simulink model "Fig134"  (R2014a)
settings: Solver=FixedStepDiscrete  StartTime=0.0  StopTime=.05  FixedStep=1.25e-6  RelTol=1e-3
undefined symbols (not defined in the file): fdesignblkfcn, gcbh
libraries: commchan3 x1, commanapbnd3 x1
(part 1 of 2)
settings Model: Creator=Dennis Silage  LastModifiedBy=Silage
settings SolverCC: AutoInsertRateTranBlk=on
settings DataIOCC: SignalLoggingSaveFormat=ModelDataLogs
settings OptimizationCC: ExpressionDepthLimit=2147483647  InitFltsAndDblsToZero=on
settings DebuggingCC: UnderspecifiedInitializationDetection=Classic  FcnCallInpInsideContextMsg=UseLocalSettings  StateNameClashWarn=warning
settings GRTTargetCC: CombineOutputUpdateFcns=off  GRTInterface=on

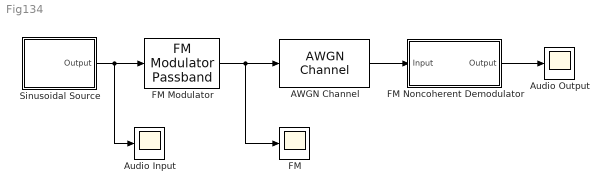
== system Fig134 ==
  AWGN Channel : commchan3/AWGN Channel  InputProcessing=Inherited (this choice will be removed - see release notes)  seed=randseed  noiseMode=Variance from mask  EbNodB=10  EsNodB=10  SNRdB=10  bitsPerSym=1  Ps=1  Tsym=1  variance=0
  Audio Output : Scope
      settings: TimeRange=0.01  MaxDataPoints=8000
  Audio Input : Scope
      settings: TimeRange=0.01  YMin=-2  YMax=2  SaveName=ScopeData2  MaxDataPoints=8000
  FM : Scope
      settings: TimeRange=0.01  MaxDataPoints=8000
  FM Modulator : commanapbnd3/FM Modulator Passband  Fc=20000  Ph=0  Kc=500
  FM Noncoherent Demodulator : Subsystem
  Sinusoidal Source : Subsystem
  wires:
  FM Noncoherent Demodulator/1(Output) -> Audio Output/1
  AWGN Channel/1 -> FM Noncoherent Demodulator/1(Input)
  Sinusoidal Source/1(Output) -> FM Modulator/1, Audio Input/1
  FM Modulator/1 -> FM/1, AWGN Channel/1

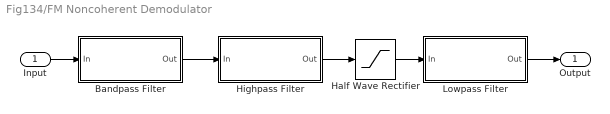
== system Fig134/FM Noncoherent Demodulator ==
  Input : Inport
  Bandpass Filter : Subsystem  DialogController=fdesignblkfcn  InitFcn=fdesignblkfcn(gcbh, {'InitFcn'});  mask(Bandpass Filter){}
      mask help: Design a bandpass filter
      settings: CopyFcn=fdesignblkfcn(gcbh, {'CopyFcn'});
      mask Help: helpview(mapfilelocation('dsp'), 'dspbandpassfilter');
      mask Display: disp('Bandpass');
  Half Wave Rectifier : Saturate  UpperLimit=2000  LowerLimit=0
  Highpass Filter : Subsystem  DialogController=fdesignblkfcn  InitFcn=fdesignblkfcn(gcbh, {'InitFcn'});  mask(Highpass Filter){}
      mask help: Design a highpass filter
      settings: CopyFcn=fdesignblkfcn(gcbh, {'CopyFcn'});
      mask Help: helpview(mapfilelocation('dsp'), 'dsphighpassfilter');
      mask Display: disp('Highpass')
  Lowpass Filter : Subsystem  DialogController=fdesignblkfcn  InitFcn=fdesignblkfcn(gcbh, {'InitFcn'});  mask(Lowpass Filter){}
      mask help: Design a lowpass filter
      settings: CopyFcn=fdesignblkfcn(gcbh, {'CopyFcn'});
      mask Help: helpview(mapfilelocation('dsp'), 'dsplowpassfilter');
      mask Display: disp('Lowpass')
  Output : Outport
  wires:
  Input/1 -> Bandpass Filter/1(In)
  Lowpass Filter/1(Out) -> Output/1
  Bandpass Filter/1(Out) -> Highpass Filter/1(In)
  Highpass Filter/1(Out) -> Half Wave Rectifier/1
  Half Wave Rectifier/1 -> Lowpass Filter/1(In)

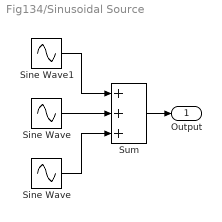
== system Fig134/Sinusoidal Source ==
  " Sine Wave " : Sin  Amplitude=0.2  Frequency=5000*pi  SampleTime=1.25e-6
  "Sine Wave " : Sin  Amplitude=0.5  Frequency=3000*pi  SampleTime=1.25e-6
  Sine Wave1 : Sin  Frequency=1000*pi  SampleTime=1.25e-6
  Sum : Sum  Inputs=+++
  Output : Outport
  wires:
  "Sine Wave "/1 -> Sum/2
  " Sine Wave "/1 -> Sum/3
  Sine Wave1/1 -> Sum/1
  Sum/1 -> Output/1

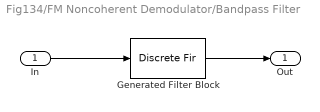
== system Fig134/FM Noncoherent Demodulator/Bandpass Filter ==
  In : Inport
  Generated Filter Block : DiscreteFir  Tag=BlockMethodSubSystem  Coefficients=[-0.00059219193775899236 -3.9341354639696544e-05 -9.7373474128287511e-05 -0.00017736431375222489 -0.00026084609867440677 -0.00032806948725862375 -0.00036584370866648712 -0.00036691313773533205 -0.00033370072449522692 -0.00027319008888497287 -0.00019739952351056374 -0.0001163690580661134 -3.9140781222203689e-05 3.181099127450536e-05 9.6227539820905477e-05 0.00016000023794347871 0.00022763267719288181 0.00030303871675504154 0.00039091787696974868 0.00048765967107231636 0.00058855101136691141 0.00068649534623964554 0.00077319127854593773 0.00084099740009888405 0.00088346211104977181 0.00089721303795390456 0.00088098366837014049 0.00083627064365611903 0.00076520196046734224 0.00067080141851764464 0.00055527961176036469 0.0004205640827085174 0.00026812716107302195 9.9654104107159327e-05 -8.383444701246304e-05 -0.00027825854448910119 -0.0004805090739020157 -0.00068454253064787786 -0.00088447748327879442 -0.0010722846019481644 -0.001241210563641256 -0.0013837332554714962 -0.0014946136234015464 -0.0015685518415167841 -0.0016029099423251838 -0.0015950876785521719 -0.0015450588833970616 -0.001452387129258103 -0.0013192212461272815 -0.0011467951995296484 -0.00093891474006392594 -0.00069926794943689667 -0.00043343301094481851 -0.00014719504052124101 0.00015162373954833613 0.00045549162478963391 0.00075535446987171377 0.0010429815127735425 0.0013091813140520443 0.00154631583251653 0.0017465737657337151 0.0019043687693183859 0.0020143886418705044 0.0020737378810482543 0.0020801006040373242 0.0020333706990985391 0.0019343178851840941 0.0017859833223153299 0.0015918143355942921 0.0013577769401517544 0.0010900122865453396 0.00079674729519155186 0.00048598940491641982 0.00016738275813494528 -0.00015022478031766337 -0.00045705470853456753 -0.00074479811325042951 -0.0010048409018170736 -0.0012305735393033264 -0.0014156419249864406 -0.001556214783327908 -0.001648896646568329 -0.001693242200470421 -0.0016891401868767324 -0.0016393031009968974 -0.0015469143446504006 -0.0014176034468437345 -0.001257098521157041 -0.0010731707335613937 -0.00087321391961068292 -0.00066604787612609595 -0.00045946941204797398 -0.00026206602515773975 -8.0763974591876357e-05 7.7355159322370164e-05 0.00020752550954445054 0.00030530870584873397 0.0003688807633016152 0.00039713463000742107 0.00039148733865793832 0.0003541714995820479 0.00028987653178021475 0.00020369688142858708 0.00010280637845851549 -5.666668614455017e-06 -0.00011312528034775884 -0.00021173410766289389 -0.00029294025870966843 -0.00034967092192513509 -0.00037487339775808001 -0.00036364294285492701 -0.00031175572978192802 -0.00021757028274392332 -8.0570566028645581e-05 9.6848944283325759e-05 0.00031116561800488118 0.00055587624105303275 0.00082363881102158725 0.001104624157779256 0.0013886456719248992 0.0016636950122589722 0.001918216905529749 0.0021397414317879003 0.0023171526333200911 0.0024393570731919461 0.0024975491552667803 0.0024838477903674503 0.0023934680182427139 0.0022231692650925006 0.0019733957296209186 0.0016464625846307887 0.0012484543176436414 0.00078736945084628175 0.00027459720599570971 -0.00027701710108238254 -0.00085186732067351007 -0.0014337446584844812 -0.002004718833691813 -0.0025473469053719526 -0.0030436349256163127 -0.0034772987448643258 -0.003832764232216063 -0.0040973477330016614 -0.0042601512492633203 -0.0043140475011803573 -0.0042545212834629396 -0.0040812808174208685 -0.0037969849215932702 -0.0034086068644421652 -0.0029258168176889161 -0.0023621924228326295 -0.0017333382604400689 -0.0010578071104098666 -0.00035507096378741899 0.00035370075965221221 0.0010477798370865531 0.0017062218335936658 0.0023099827226738204 0.0028412269206391084 0.0032852975051397156 0.0036299328235587392 0.003867053497780893 0.0039916497646677465 0.004003411793243445 0.0039052810333668293 0.0037047539842970014 0.0034122442742909784 0.0030420102713529097 0.0026102665367740887 0.0021358806009585413 0.0016383152462557235 0.001138134065413366 0.00065488315748309166 0.00020758667295421894 ...(+7989 chars)]  InputProcessing=Columns as channels (frame based)
  Out : Outport
  wires:
  In/1 -> Generated Filter Block/1
  Generated Filter Block/1 -> Out/1

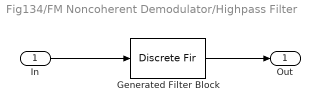
== system Fig134/FM Noncoherent Demodulator/Highpass Filter ==
  In : Inport
  Generated Filter Block : DiscreteFir  Tag=BlockMethodSubSystem  Coefficients=[0.14605653992459219 0.0018324539324470757 0.00078039104697391615 -0.00081843411535514887 -0.0032722829557158828 -0.0064608348125574089 -0.010681720440550657 -0.015920677165552927 -0.02263431673035754 -0.031094309724005557 -0.042293482298376608 -0.057593757192581536 -0.080550142915381859 -0.11974631073735834 -0.20775174708812086 -0.63532020255695199 0.63532020255695199 0.20775174708812086 0.11974631073735834 0.080550142915381859 0.057593757192581536 0.042293482298376608 0.031094309724005557 0.02263431673035754 0.015920677165552927 0.010681720440550657 0.0064608348125574089 0.0032722829557158828 0.00081843411535514887 -0.00078039104697391615 -0.0018324539324470757 -0.14605653992459219]  InputProcessing=Columns as channels (frame based)
  Out : Outport
  wires:
  Generated Filter Block/1 -> Out/1
  In/1 -> Generated Filter Block/1
